simulink model "IdealGen_load_CtrlGen_wWT_abc_detailed"  (R2023b)
settings: Solver=VariableStepAuto  StartTime=0.0  StopTime=Tend  RelTol=1e-3
undefined symbols (not defined in the file): C_dc, c_drt, C_f, C_p_opt, f_nom, H_gen, H_vsm, H_WTR, I_dc_base, Ibase_hv, Ibase_lv, k_d_vsm, k_drt, k_p_p_vsm, k_p_q_vsm, K_pitch, Ki_cc, ki_q, Ki_vc, Kp_cc, Kp_vc, L_d, l_f, L_f, L_grid, L_mv, L_q, l_t_hvmv, l_t_mvlv, lambda_opt, Lbase1v, omega_nom, omega_WTR_min, omega_WTR_n, omega_WTR_sl, phase_shift_test_state, phase_shifts, pitch_max, pitch_min, Pitchanglevector, Pmax, Powercoefficient, psi_pm, R_a, r_f, R_grid, R_mv, r_t_hvmv, r_t_mvlv, R_WTR, rate_max, rate_min, rocof_slope, Rocof_test_state, Sbase1, Sbase_t1, T_base, T_pitch, T_servo, Tchange_gfm_ref ... (+12)
libraries: spsControlledVoltageSourceLib x6, slpidlib x6, spsPower3phInstantaneousLib x4, spsThreePhaseSeriesRLCBranchLib x4, spsCurrentMeasurementLib x3, spsThreePhaseVIMeasurementLib x3, spsRMSLib x3, spsabctodq0Lib x3, spsGroundLib x2, spsdq0toabcLib x2, spsSeriesRLCBranchLib x2, spsVoltageMeasurementLib x2
(part 1 of 2)
settings Model: Creator=s183702  LastModifiedBy=Martin Pedersen
settings HardwareCC: ProdBitPerLong=64  ProdLargestAtomicFloat=None  ProdHWDeviceType=AMD->Athlon 64

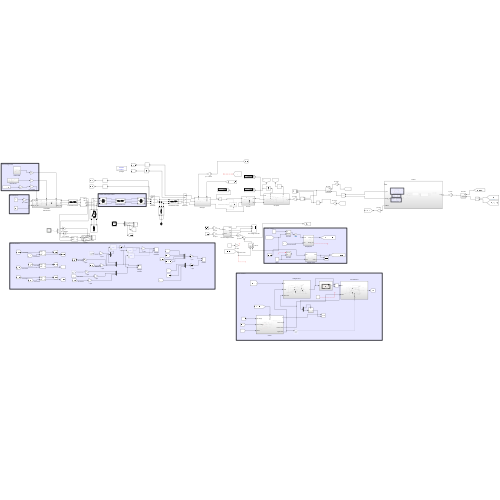
[thumbnail: Simulink's stored preview of the top-level diagram]
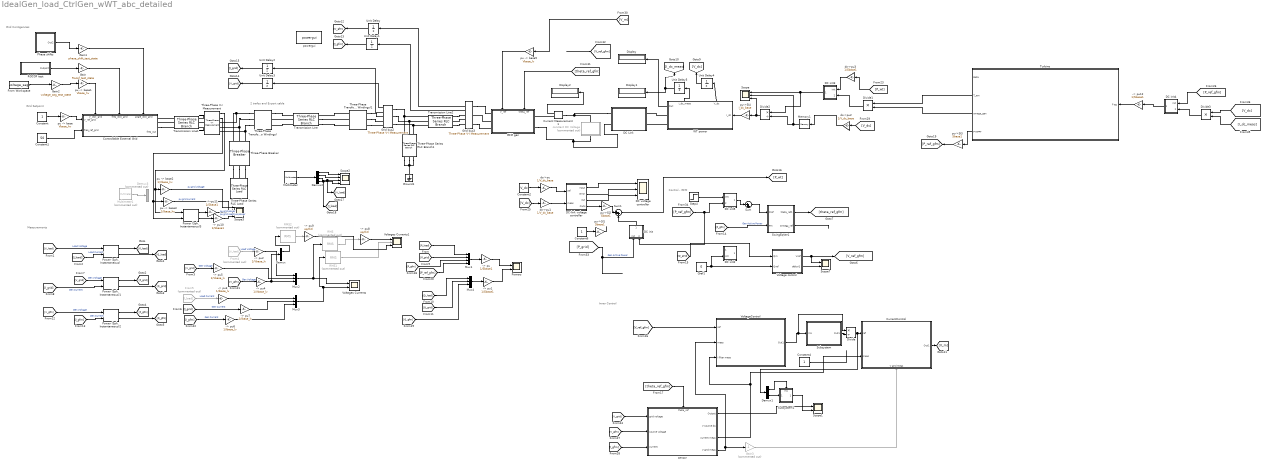
== system IdealGen_load_CtrlGen_wWT_abc_detailed ==
  note: Inner Control
  note: Grid Setpoint
  note: Grid Contigencies
  note: Control - GFM
  note: Measurements
  note: 2 trafos and Export cable
  -> pu{,1,10..12} (5 alike) : Gain  Gain=1/Sbase1
  -> pu2 : Gain  Gain=1/Vbase_lv
  -> pu3 : Gain  Gain=1/Ibase_lv
  -> pu4 : Gain  Gain=1/Vbase_lv
  -> pu5 : Gain  Gain=1/Vbase_lv
  -> pu6 : Gain  Gain=1/Ibase_lv
  -> pu7 : Gain  Gain=1/Ibase_lv
  -> pu8 : Gain  Gain=sqrt(2)
  -> pu9 : Gain  Gain=sqrt(2)
  Constant : Constant
  Constant1 : Constant  Value=50
  Constant2 : Constant  Value=V_dc
  Constant4 : Constant
  Constant6 : Constant
  Controllable External Grid : Subsystem
      settings: PortSchema="{\"entries\":[{\"content\":{\"sides\":[{\"content\":{\"connectorIds\":[\"In1\",\"In2\"]},\"type\":\"ConnectorPlacement.EquallySpacedRectSide\",\"uuid\":\"c82e3ee4-47de-4631-9682-a189e406d2fd\"},{\"content\":{\"connectorIds\":[\"RConn1\",\"RConn2\",\"RConn3\",\"Out1\"],\"side\":\"RIGHT\"},\"type\":\"ConnectorPlacement.EquallySpacedRectSide\",\"uuid\":\"b806e225-811d-4112-8c3d-45e9b8086e84\"},{\"content\":{\"connectorIds\":[\"In3\",\"In4\",\"In5\"],\"side\":\"TOP\"},\"type\":\"ConnectorPlacement.EquallySpacedRectSide\",\"uuid\":\"c79b677b-bc74-4454-b0f0-10f0f27e0767\"}]},\"type\":\"ConnectorPlacement.EquallySpacedConnector\",\"uuid\":\"44354c03-b4f0-403a-803b-b669dc1296a6\"}],\"packageUris\":[\"http://schema.mathworks.com/mf0/Connector/R2020b\"],\"version\":\"1.0\"}"
  Current Measurement1 : spsCurrentMeasurementLib/Current Measurement  PhasorSimulation=off  OutputType=Complex  PSBequivalent=0
  CurrentControl : Subsystem
      settings: PortSchema="{\"entries\":[{\"content\":{\"sides\":[{\"content\":{\"connectorIds\":[\"In1\",\"In2\"]},\"type\":\"ConnectorPlacement.EquallySpacedRectSide\",\"uuid\":\"219db9ea-637c-42c0-b87e-0a8373949a2f\"},{\"content\":{\"connectorIds\":[\"Out1\"],\"side\":\"RIGHT\"},\"type\":\"ConnectorPlacement.EquallySpacedRectSide\",\"uuid\":\"817edf77-a627-4761-8536-4c41ccdce557\"},{\"content\":{\"side\":\"TOP\"},\"type\":\"ConnectorPlacement.EquallySpacedRectSide\",\"uuid\":\"b4d64eff-9104-48e3-a4e2-ec81b224adc3\"},{\"content\":{\"connectorIds\":[\"In3\"],\"side\":\"BOTTOM\"},\"type\":\"ConnectorPlacement.EquallySpacedRectSide\",\"uuid\":\"8db682a6-86bb-4d51-9cc3-8f643a502240\"}]},\"type\":\"ConnectorPlacement.EquallySpacedConnector\",\"uuid\":\"cfbf309f-cee6-401c-8c28-748b4359d9c9\"}],\"packageUris\":[\"http://schema.mathworks.com/mf0/Connector/R2020b\"],\"version\":\"1.0\"}"
  DC Link : Subsystem
  DC init : Subsystem
  DC init2 : Subsystem
  DC init3 : Subsystem
  DC init4 : Subsystem
  DC init5 : Subsystem
  DC voltage controller : Scope  NumInputPorts=3
  DC-link voltage controller : Subsystem
  Demux : Demux  Outputs=3
  Demux1 : Demux  Outputs=2
  Demux2 : Demux
  Demux3 : Demux  Commented=on  Outputs=2
  Display : Display
  Display1 : Display
  Display2 : Display
  Divide : Product  Inputs=*/
  Divide1 : Product  Inputs=**
  Divide2 : Product  Inputs=*/
  Divide3 : Product  Inputs=**
  From Workspace : FromWorkspace  VariableName=voltage_sags
  From4 : From  Commented=on  GotoTag=V_load  TagVisibility=global
  From5 : From  Commented=on  GotoTag=I_load
  GFM gen : Subsystem
      settings: PortSchema="{\"entries\":[{\"content\":{\"sides\":[{\"content\":{\"connectorIds\":[\"LConn1\",\"LConn2\"]},\"type\":\"ConnectorPlacement.EquallySpacedRectSide\",\"uuid\":\"b9b898d8-aa2c-4fc0-879f-33950e845205\"},{\"content\":{\"connectorIds\":[\"RConn1\",\"RConn2\",\"RConn3\"],\"side\":\"RIGHT\"},\"type\":\"ConnectorPlacement.EquallySpacedRectSide\",\"uuid\":\"0f5f2870-ceda-40eb-961f-274893a00dd5\"},{\"content\":{\"connectorIds\":[\"In1\",\"In2\"],\"side\":\"TOP\"},\"type\":\"ConnectorPlacement.EquallySpacedRectSide\",\"uuid\":\"16b0f3cd-2bcf-4c98-bcc9-1e9131637ccf\"}]},\"type\":\"ConnectorPlacement.EquallySpacedConnector\",\"uuid\":\"5f5ec50b-7fca-4ced-b434-e49ba9676af4\"}],\"packageUris\":[\"http://schema.mathworks.com/mf0/Connector/R2020b\"],\"version\":\"1.0\"}"
  Gain : Gain  Gain=Rocof_test_state
  Gain1 : Gain  Gain=phase_shift_test_state
  Gain2 : Gain  Gain=voltage_sag_test_state
  Gain3 : Gain  Commented=on  Gain=-1
  Grid bus2 : spsThreePhaseVIMeasurementLib/Three-Phase V-I Measurement  VoltageMeasurement=phase-to-ground  SetLabelV=off  LabelV=V_grid  Vpu=off  VpuLL=off  CurrentMeasurement=yes  SetLabelI=off  LabelI=I_grid  Ipu=off  Pbase=100e6  Vbase=500e3  OutputType=Complex  PhasorSimulation=off  PSBequivalent=0
  Grid bus3 : spsThreePhaseVIMeasurementLib/Three-Phase V-I Measurement  VoltageMeasurement=phase-to-ground  SetLabelV=off  LabelV=V_gfm  Vpu=off  VpuLL=off  CurrentMeasurement=yes  SetLabelI=off  LabelI=I_gfm  Ipu=off  Pbase=100e6  Vbase=500e3  OutputType=Complex  PhasorSimulation=off  PSBequivalent=0
  Ground1 : spsGroundLib/Ground  LConnTagsString=a
  Memory1 : Memory  InitialCondition=1
  Multimeter : spsMultimeterLib/Multimeter  L=21  sel=[7 8 9 19 20 21 4 5 6 16 17 18]  yselected={}  Gain=[1 1 1 1 1 1 1 1 1 1 1 1]  OutputType=Complex  PlotAtSimulationStop=off  PhasorSimulation=off
  Multimeter1 : spsMultimeterLib/Multimeter  Commented=on  L=21  sel=[7 8 9 13 14 15]  yselected={}  Gain=[1 1 1 1 1 1]  OutputType=Complex  PlotAtSimulationStop=off  PhasorSimulation=off
  Mux1 : Mux
  Mux2 : Mux  Inputs=3
  Mux3 : Mux  Inputs=3
  Mux4 : Mux  Inputs=3
  Phase shifts : Subsystem
  Power (3ph, Instantaneous){,1..3} (4 alike) : spsPower3phInstantaneousLib/Power (3ph, Instantaneous)
  Powers : Scope  NumInputPorts=2
  Qref1 : Constant  Value=0
  RMS : spsRMSLib/RMS  Commented=on  TrueRMS=on  Freq=50  RMSInit=1  Ts=0
  RMS1 : spsRMSLib/RMS  Commented=on  TrueRMS=on  Freq=50  RMSInit=1  Ts=0
  RMS2 : spsRMSLib/RMS  Commented=on  TrueRMS=on  Freq=50  RMSInit=1  Ts=0
  ROCOF test : Subsystem
  Scope : Scope  NumInputPorts=3
  Scope1 : Scope  NumInputPorts=2
  Scope2 : Scope  NumInputPorts=4
  Scope3 : Scope  NumInputPorts=4
  Scope7 : Scope  NumInputPorts=2
  Step4 : Step  Time=Tchange_gfm_ref  Before=Sbase1*0.4  After=Sbase1*0.4  SampleTime=0
  Subsystem : Subsystem
  Subsystem1 : Subsystem
      settings: PortSchema="{\"entries\":[{\"content\":{\"sides\":[{\"content\":{\"connectorIds\":[\"In1\"]},\"type\":\"ConnectorPlacement.EquallySpacedRectSide\",\"uuid\":\"4a76dc79-b416-43cf-afab-f92cfdf0ce39\"},{\"content\":{\"connectorIds\":[\"Out1\"],\"side\":\"RIGHT\"},\"type\":\"ConnectorPlacement.EquallySpacedRectSide\",\"uuid\":\"95d72f6b-ef09-433d-aae0-c8341f391507\"},{\"content\":{\"connectorIds\":[\"In2\"],\"side\":\"TOP\"},\"type\":\"ConnectorPlacement.EquallySpacedRectSide\",\"uuid\":\"0145e476-49d1-4b43-865a-36bbad1700d0\"}]},\"type\":\"ConnectorPlacement.EquallySpacedConnector\",\"uuid\":\"1d1114a5-8d57-4d93-ab19-43d07f54280a\"}],\"packageUris\":[\"http://schema.mathworks.com/mf0/Connector/R2020b\"],\"version\":\"1.0\"}"
  Sum : Sum  Inputs=|++
  Sum1 : Sum  Inputs=|++
  SwingEqVer1 : Subsystem
  Three-Phase Series RLC Branch1 : spsThreePhaseSeriesRLCBranchLib/Three-Phase Series RLC Branch  LConnTagsString=A|B|C  RConnTagsString=A|B|C  BranchType=C  Resistance=0.001*Zbase1v  Inductance=L_f  Capacitance=C_f  Measurements=Branch currents
  Three-Phase Series RLC Load : spsThreePhaseSeriesRLCLoadLib/Three-Phase Series RLC Load  LConnTagsString=A|B|C  Configuration=Y (grounded)  NominalVoltage=Vbase_hv*sqrt(3/2)  Vabc=[1e3 1e3 1e3]  Vabcp=[1e3 1e3 1e3]  NominalFrequency=50  UnbalancedPower=off  ActivePower=Sbase1*0.5  InductivePower=0  CapacitivePower=0  Pabc=[10e3 9e3 11e3]  QLabc=[100 90 110]  QCabc=[100 90 110]  Pabcp=[10e3 9e3 11e3]  QLabcp=[100 90 110]  QCabcp=[100 90 110]  Measurements=Branch voltages and currents  LoadType=constant Z
  Three-Phase Transformer (Two Windings) : spsThreePhaseTransformerTwoWindingsLib/Three-Phase Transformer (Two Windings)  Winding1Connection=Yg  Winding2Connection=Yg  CoreType=Three single-phase transformers  SetSaturation=off  Hysteresis=off  DataFile='hysteresis'  SetInitialFlux=off  Measurements=None  UNITS=pu  NominalPower=[ Sbase1 , f_nom ]  Winding1=[ Vbase_hv*sqrt(3/2) , r_t_hvmv/2 , l_t_hvmv/2]  Winding2=[ Vbase_mv*sqrt(3/2) , r_t_hvmv/2, l_t_hvmv/2 ]  Rm=500  Lm=500  L0=0.5  Saturation=[ 0,0 ; 0.0024,1.2 ; 1.0,1.52 ]  InitialFluxes=[ 0.8 , -0.8 , 0.7 ]  BreakLoop=off  DiscreteSolver=Trapezoidal iterative  DataType=off  TransfoNumber=1
  Three-Phase Transformer (Two Windings)1 : spsThreePhaseTransformerTwoWindingsLib/Three-Phase Transformer (Two Windings)  Winding1Connection=Yg  Winding2Connection=Yg  CoreType=Three single-phase transformers  SetSaturation=off  Hysteresis=off  DataFile='hysteresis'  SetInitialFlux=off  Measurements=None  UNITS=pu  NominalPower=[ Sbase_t1 , f_nom ]  Winding1=[ Vbase_mv*sqrt(3/2) , r_t_mvlv/2 , l_t_mvlv/2]  Winding2=[ Vbase_lv*sqrt(3/2) , r_t_mvlv/2, l_t_mvlv/2 ]  Rm=500  Lm=500  L0=0.5  Saturation=[ 0,0 ; 0.0024,1.2 ; 1.0,1.52 ]  InitialFluxes=[ 0.8 , -0.8 , 0.7 ]  BreakLoop=off  DiscreteSolver=Trapezoidal iterative  DataType=off  TransfoNumber=1
  Three-Phase V-I Measurement : spsThreePhaseVIMeasurementLib/Three-Phase V-I Measurement  VoltageMeasurement=phase-to-ground  SetLabelV=off  LabelV=Vabc  Vpu=off  VpuLL=off  CurrentMeasurement=yes  SetLabelI=off  LabelI=Iabc  Ipu=off  Pbase=100e6  Vbase=500e3  OutputType=Complex  PhasorSimulation=off  PSBequivalent=0
  Three-Phase Breaker : spsThreePhaseBreakerLib/Three-Phase Breaker  InitialState=open  SwitchA=on  SwitchB=on  SwitchC=on  SwitchTimes=[30]  External=off  BreakerResistance=0.01  SnubberResistance=1e6  SnubberCapacitance=inf  Measurements=Breaker voltages and currents
  Transmission Line : spsThreePhaseSeriesRLCBranchLib/Three-Phase Series RLC Branch  LConnTagsString=A|B|C  RConnTagsString=A|B|C  BranchType=RL  Resistance=R_mv  Inductance=L_mv  Capacitance=0  Measurements=None
  Transmission Line1 : spsThreePhaseSeriesRLCBranchLib/Three-Phase Series RLC Branch  LConnTagsString=A|B|C  RConnTagsString=A|B|C  BranchType=RL  Resistance=R_grid  Inductance=L_grid  Capacitance=0  Measurements=Branch voltages and currents
  Transmission Line2 : spsThreePhaseSeriesRLCBranchLib/Three-Phase Series RLC Branch  LConnTagsString=A|B|C  RConnTagsString=A|B|C  BranchType=RL  Resistance=r_f*Zbase1v  Inductance=l_f*Lbase1v  Capacitance=0  Measurements=None
  Turbine : Subsystem
  Unit Delay{,1..3,5} (5 alike) : UnitDelay  SampleTime=-1  HasFrameUpgradeWarning=on
  Unit Delay4 : UnitDelay  InitialCondition=V_dc  SampleTime=-1  HasFrameUpgradeWarning=on
  Voltage control : Subsystem
  VoltageControl : Subsystem
  Voltages Currents : Scope  NumInputPorts=2
  Voltages Currents1 : Scope  NumInputPorts=3
  WT power : Subsystem
      settings: PortSchema="{\"entries\":[{\"content\":{\"sides\":[{\"content\":{\"connectorIds\":[\"In1\"]},\"type\":\"ConnectorPlacement.EquallySpacedRectSide\",\"uuid\":\"9d3e38d2-6add-483d-9a31-3b5598dff8d3\"},{\"content\":{\"connectorIds\":[\"Out1\",\"RConn1\",\"RConn2\"],\"side\":\"RIGHT\"},\"type\":\"ConnectorPlacement.EquallySpacedRectSide\",\"uuid\":\"7ce5d226-07b0-4d85-bacd-eba224635451\"},{\"content\":{\"connectorIds\":[\"Out2\",\"Out3\"],\"side\":\"TOP\"},\"type\":\"ConnectorPlacement.EquallySpacedRectSide\",\"uuid\":\"1864accd-580c-4e01-b41e-4bc1921d0b77\"},{\"content\":{\"side\":\"BOTTOM\"},\"type\":\"ConnectorPlacement.EquallySpacedRectSide\",\"uuid\":\"0a771f6d-f5fb-412d-b2d7-9d95c39f39de\"}]},\"type\":\"ConnectorPlacement.EquallySpacedConnector\",\"uuid\":\"874bd654-abb7-47d1-80fe-1eaf36f4fe8a\"}],\"packageUris\":[\"http://schema.mathworks.com/mf0/Connector/R2020b\"],\"version\":\"1.0\"}"
  constant DC Voltage : Subsystem  Commented=on
  dc->pu : Gain  Gain=1/V_dc_base
  dc->pu1 : Gain  Gain=1/V_dc_base
  dc->pu2 : Gain  Gain=1/V_dc_base
  dc->pu3 : Gain  Gain=1/Sbase1
  powergui : sps_lib/powergui  Priority=1  SimulationMode=Discrete  SampleTime=5e-6  frequency=60  Iterations=50  frequencyindice=0  Pbase=100e6  ErrMax=1e-4  UnitsV=kV  UnitsW=MW  buscounter=0  FunctionMessages=off  echomessages=off  EnableUseOfTLC=off  CurrentSourceSwitches=off  DisableSnubberDevices=off  DisableRonSwitches=off  DisableVfSwitches=off  DisplayEquations=off  AutomaticDiscreteSolvers=off  SolverType=Tustin/Backward Euler (TBE)  Interpol=off  ExternalGateDelay=off  methode=off  Ts=100  x0status=blocks  SPID=on  SwTol=0  HookPort=off  NonlinearTolerance=1e-4  nMaxIteration=100  ContinueOnMaxIteration=off  RestoreLinks=warning  ResistiveCurrentMeasurement=off  Frange=[0:2:500]  Ylog=off  Xlog=on  ShowGrid=off  save=off  variable=ZData  structure=0  ZoomFFT=off  StartTime=0.0  cycles=1  DisplayStyle=1  fundamental=60  FreqAxis=off  MaxFrequency=1000  frequencyindicesteady=1  RmsSteady=1  display=off
  "pu -> base" : Gain  Gain=Vbase_hv
  "pu -> base1" : Gain  Gain=Vbase_hv
  "pu -> base2" : Gain  Gain=1/Vbase_hv
  "pu -> base3" : Gain  Gain=1/Ibase_hv
  "pu -> base5" : Gain  Gain=Vbase_lv
  pu->SI1 : Gain  Gain=Sbase1
  pu->SI2 : Gain  Gain=Sbase1
  pu->SI3 : Gain  Gain=Sbase1
  pu->SI4 : Gain  Gain=I_dc_base
  sensor : Subsystem
      settings: PortSchema="{\"entries\":[{\"content\":{\"sides\":[{\"content\":{\"connectorIds\":[\"In1\",\"In2\",\"In3\"]},\"type\":\"ConnectorPlacement.EquallySpacedRectSide\",\"uuid\":\"f6076434-f402-4e41-b507-98b228e724d5\"},{\"content\":{\"connectorIds\":[\"Out1\",\"Out2\",\"Out3\",\"Out4\"],\"side\":\"RIGHT\"},\"type\":\"ConnectorPlacement.EquallySpacedRectSide\",\"uuid\":\"ad78b019-92bf-45d4-be49-d5eeb6323d07\"},{\"content\":{\"side\":\"TOP\"},\"type\":\"ConnectorPlacement.EquallySpacedRectSide\",\"uuid\":\"9dc9234e-7a1d-4b97-8830-6d3adbb504ce\"},{\"content\":{\"connectorIds\":[\"In4\"],\"side\":\"BOTTOM\"},\"type\":\"ConnectorPlacement.EquallySpacedRectSide\",\"uuid\":\"085a8b4b-0a39-42f8-9e4d-5287113458ab\"}]},\"type\":\"ConnectorPlacement.EquallySpacedConnector\",\"uuid\":\"c1a424bf-dbfe-42ba-bd00-ed441f443675\"}],\"packageUris\":[\"http://schema.mathworks.com/mf0/Connector/R2020b\"],\"version\":\"1.0\"}"
  wires:
  From5/1 -> -> pu3/1  "Load Current"
  From4/1 -> -> pu2/1  "Load Voltage"
  [V_grid] -> -> pu5/1  "Gen Voltage"
  [I_grid] -> -> pu7/1  "Gen Current"
  "pu -> base"/1 -> Controllable External Grid/1(V_ref_grid)
  Constant/1 -> "pu -> base"/1
  Constant1/1 -> Controllable External Grid/2(freq_ref_grid)
  Gain2/1 -> "pu -> base1"/1
  ROCOF test/1(Outport) -> Gain/1
  "pu -> base1"/1 -> Controllable External Grid/3(V_dist_grid)
  [V_load] -> "Power (3ph, Instantaneous)"/1  "Load Voltage"
  [I_load] -> "Power (3ph, Instantaneous)"/2  "Load Current"
  [V_grid] -> "Power (3ph, Instantaneous)1"/1  "Gen Voltage"
  [I_grid] -> "Power (3ph, Instantaneous)1"/2  "Gen Current"
  "Power (3ph, Instantaneous)"/1 -> [P_load]
  "Power (3ph, Instantaneous)"/2 -> [Q_load]
  "Power (3ph, Instantaneous)1"/1 -> [P_grid]
  "Power (3ph, Instantaneous)1"/2 -> [Q_grid]
  [Q_load] -> Mux4/1
  [Q_grid] -> Mux4/2
  [P_grid] -> Mux1/2
  [P_load] -> Mux1/1
  Mux4/1 -> -> pu1/1
  Mux1/1 -> -> pu/1
  -> pu/1 -> Powers/1
  -> pu1/1 -> Powers/2
  "pu -> base5"/1 -> GFM gen/2(V_ref)
  "Power (3ph, Instantaneous)2"/2 -> [Q_gfm]
  "Power (3ph, Instantaneous)2"/1 -> [P_gfm]
  [I_gfm] -> "Power (3ph, Instantaneous)2"/2  "Gen Current"
  [V_gfm] -> "Power (3ph, Instantaneous)2"/1  "Gen Voltage"
  [P_gfm] -> SwingEqVer1/2(Pm)  "Gen Active Power"
  SwingEqVer1/2(Omega_ref) -> ?
  SwingEqVer1/1(theta_ref1) -> [theta_ref_gfm]
  Qref1/1 -> DC init2/2(init), Voltage control/2(Qref)
  Voltage control/1(Vref) -> Scope7/1, [V_ref_gfm]
  Voltage control/2(delta Q) -> Scope7/2
  ? -> DC init2/1(second)
  [V_ref_gfm] -> ?
  [theta_ref_gfm] -> GFM gen/1(theta_ref)
  [P_gfm] -> Mux1/3
  [Q_gfm] -> Mux4/3
  [P_ref_gfm] -> Mux1/4
  [V_gfm] -> -> pu4/1  "Gen Voltage"
  [I_gfm] -> -> pu6/1  "Gen Current"
  Mux2/1 -> RMS/1, Voltages Currents/1
  Mux3/1 -> RMS1/1, Voltages Currents/2
  -> pu2/1 -> Mux2/1
  -> pu4/1 -> Demux/1, Mux2/3
  -> pu5/1 -> Mux2/2
  -> pu3/1 -> Mux3/1
  -> pu6/1 -> Mux3/3
  RMS/1 -> -> pu8/1
  RMS1/1 -> Voltages Currents1/2
  -> pu7/1 -> Mux3/2
  -> pu8/1 -> Voltages Currents1/1
  RMS2/1 -> -> pu9/1
  -> pu9/1 -> Voltages Currents1/3
  Demux/1 -> RMS2/1
  WT power/2(V_dc) -> Unit Delay4/1
  WT power/1(Pwt) -> Display/1
  Constant2/1 -> dc->pu/1
  [V_dc] -> dc->pu1/1
  DC-link voltage controller/1(input) -> DC voltage controller/1
  DC-link voltage controller/2(error) -> DC voltage controller/2
  DC-link voltage controller/3(out) -> DC voltage controller/3
  WT power/3(i_dc_meas) -> Unit Delay5/1
  Divide1/1 -> DC init3/2(second)
  Memory1/1 -> Scope/2, Divide2/2
  Divide2/1 -> Scope/3, pu->SI4/1
  dc->pu/1 -> DC-link voltage controller/1(ref)
  dc->pu1/1 -> DC-link voltage controller/2(meas)
  Gain/1 -> Controllable External Grid/4(freq_dist_grid)
  Gain1/1 -> Controllable External Grid/5(angle_dist_grid)
  Phase shifts/1(Out2) -> Gain1/1
  From Workspace/1 -> Gain2/1
  [theta_ref_gfm] -> sensor/4(theta_ref)
  [V_ref_gfm] -> VoltageControl/1(ref)
  sensor/1(V grid meas) -> VoltageControl/2(meas), Gain3/1
  sensor/2(current meas) -> VoltageControl/3(I filter meas), CurrentControl/2(meas)
  [I_gfm] -> sensor/1(current)
  [V_grid] -> sensor/3(grid voltage)
  [V_gfm] -> sensor/2(source voltage)
  CurrentControl/1(Out1) -> [V_m]
  [V_m] -> "pu -> base5"/1
  Gain3/1 -> CurrentControl/3(V grid meas)
  Divide/1 -> Demux1/1, CurrentControl/1(ref)
  VoltageControl/1(Out1) -> Divide/1, Subsystem/1(In1)
  Constant4/1 -> ?
  Grid bus3/1 -> Unit Delay/1
  Unit Delay2/1 -> [I_grid]
  Unit Delay3/1 -> [V_grid]
  Unit Delay1/1 -> [I_gfm]
  Unit Delay/1 -> [V_gfm]
  Grid bus3/2 -> Unit Delay1/1
  Grid bus2/1 -> Unit Delay3/1
  Grid bus2/2 -> Unit Delay2/1
  Unit Delay4/1 -> [V_dc]
  Unit Delay5/1 -> [I_dc_meas], Display1/1
  [V_dc] -> dc->pu2/1
  Sum/1 -> SwingEqVer1/1(Pref)
  Constant6/1 -> pu->SI1/1
  DC-link voltage controller/4(Out4) -> pu->SI2/1
  [P_grid] -> DC init/1(init)  "Gen Active Power"
  pu->SI2/1 -> Sum1/1
  Subsystem/1(Out1) -> Divide/2
  pu->SI1/1 -> ?
  sensor/4(Output) -> Scope1/1
  Subsystem1/1(Out1) -> Scope1/2
  Demux1/1 -> Subsystem1/2(In1)
  Demux1/2 -> Subsystem1/1(In2)
  Multimeter/1 -> Demux2/1
  Demux2/1 -> Scope2/1
  Demux2/2 -> Scope2/2
  Demux2/3 -> Scope2/3, [V_load]
  Demux2/4 -> [I_load], Scope2/4
  Multimeter1/1 -> Demux3/1
  Three-Phase V-I Measurement/1 -> "Power (3ph, Instantaneous)3"/1, "pu -> base2"/1
  "pu -> base2"/1 -> Scope3/1  "pu grid voltage"
  Three-Phase V-I Measurement/2 -> "Power (3ph, Instantaneous)3"/2, "pu -> base3"/1
  "pu -> base3"/1 -> Scope3/2  "pu grid current"
  "Power (3ph, Instantaneous)3"/2 -> -> pu10/1
  "Power (3ph, Instantaneous)3"/1 -> -> pu11/1
  -> pu11/1 -> Scope3/3  "pu grid power"
  -> pu10/1 -> Scope3/4  "pu grid reactive power"
  Turbine/4(P MPPT) -> pu->SI3/1
  pu->SI3/1 -> [P_ref_gfm]
  Turbine/3(omega_gen) -> Divide1/2
  [P_ref_gfm] -> DC init4/1(init)
  -> pu12/1 -> Turbine/1(P ag)
  Turbine/2(T_em) -> Divide1/1
  dc->pu2/1 -> Memory1/1
  pu->SI4/1 -> WT power/1(I_dc)
  Divide3/1 -> DC init4/2(second)
  [I_dc_meas] -> Divide3/2
  DC init3/1("   ") -> Divide2/1, Scope/1
  Current Measurement1/1 -> Display2/1
  [Q_grid] -> Voltage control/1(Qm)
  [P_ref_gfm] -> DC init5/2(second), DC init/2(second)
  Sum1/1 -> [P_wt]
  DC init4/1("   ") -> -> pu12/1
  [V_dc] -> Divide3/1
  [P_wt] -> dc->pu3/1
  DC init5/1("   ") -> Sum/1
  Step4/1 -> DC init5/1(init)
  dc->pu3/1 -> DC init3/1(init)
  DC init/1("   ") -> Sum1/2
  connections:
  Three-Phase Series RLC Branch1/LConn2 -- Grid bus2/LConn2 -- Transmission Line2/LConn2
  Three-Phase Series RLC Branch1/LConn1 -- Grid bus2/LConn1 -- Transmission Line2/LConn1
  Three-Phase Series RLC Branch1/LConn3 -- Grid bus2/LConn3 -- Transmission Line2/LConn3
  Three-Phase Transformer (Two Windings)1/RConn1 -- Grid bus2/RConn1
  Three-Phase Transformer (Two Windings)1/RConn2 -- Grid bus2/RConn2
  Three-Phase Transformer (Two Windings)1/RConn3 -- Grid bus2/RConn3
  Transmission Line1/LConn1 -- Controllable External Grid/RConn1
  Transmission Line1/LConn2 -- Controllable External Grid/RConn2
  Controllable External Grid/RConn3 -- Transmission Line1/LConn3
  GFM gen/RConn2 -- Grid bus3/LConn2
  Grid bus3/LConn1 -- GFM gen/RConn1
  Grid bus3/LConn3 -- GFM gen/RConn3
  Transmission Line2/RConn1 -- Grid bus3/RConn1
  Grid bus3/RConn2 -- Transmission Line2/RConn2
  Transmission Line2/RConn3 -- Grid bus3/RConn3
  GFM gen/LConn2 -- DC Link/LConn2 -- constant DC Voltage/RConn1
  WT power/RConn1 -- DC Link/RConn1
  WT power/RConn2 -- DC Link/RConn2
  Three-Phase Series RLC Branch1/RConn2 -- Three-Phase Series RLC Branch1/RConn1 -- Three-Phase Series RLC Branch1/RConn3 -- Ground1/LConn1
  Three-Phase Transformer (Two Windings)/RConn1 -- Transmission Line/LConn1
  Transmission Line/RConn2 -- Three-Phase Transformer (Two Windings)1/LConn2
  Transmission Line/LConn2 -- Three-Phase Transformer (Two Windings)/RConn2
  Transmission Line/RConn3 -- Three-Phase Transformer (Two Windings)1/LConn3
  Three-Phase Transformer (Two Windings)1/LConn1 -- Transmission Line/RConn1
  Transmission Line/LConn3 -- Three-Phase Transformer (Two Windings)/RConn3
  Three-Phase Transformer (Two Windings)/LConn1 -- Three-Phase V-I Measurement/RConn1 -- Three-Phase Breaker/LConn1
  Three-Phase Transformer (Two Windings)/LConn2 -- Three-Phase V-I Measurement/RConn2 -- Three-Phase Breaker/LConn2
  Three-Phase Transformer (Two Windings)/LConn3 -- Three-Phase V-I Measurement/RConn3 -- Three-Phase Breaker/LConn3
  DC Link/LConn1 -- constant DC Voltage/LConn1 -- Current Measurement1/LConn1
  Three-Phase Breaker/RConn1 -- Three-Phase Series RLC Load/LConn1
  Three-Phase Breaker/RConn2 -- Three-Phase Series RLC Load/LConn2
  Three-Phase Breaker/RConn3 -- Three-Phase Series RLC Load/LConn3
  Three-Phase V-I Measurement/LConn2 -- Transmission Line1/RConn2
  Three-Phase V-I Measurement/LConn1 -- Transmission Line1/RConn1
  Three-Phase V-I Measurement/LConn3 -- Transmission Line1/RConn3
  Current Measurement1/RConn1 -- GFM gen/LConn1

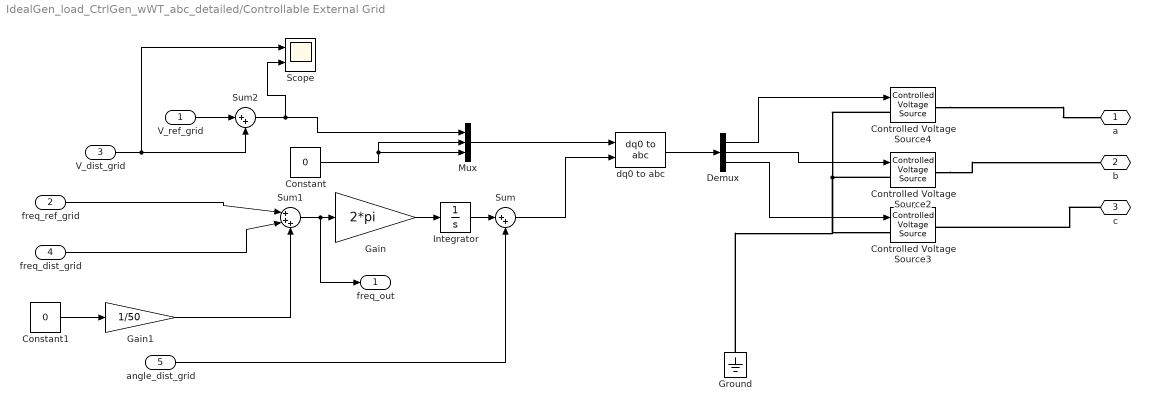
== system IdealGen_load_CtrlGen_wWT_abc_detailed/Controllable External Grid ==
  V_ref_grid : Inport
  freq_ref_grid : Inport  Port=2
  V_dist_grid : Inport  Port=3
  freq_dist_grid : Inport  Port=4
  angle_dist_grid : Inport  Port=5
  Constant : Constant  Value=0
  Constant1 : Constant  Value=0
  Controlled Voltage Source2 : spsControlledVoltageSourceLib/Controlled Voltage Source  Initialize=on  Source_Type=AC  Amplitude=Vbase_lv  Phase=-120  Frequency=50  Measurements=None
  Controlled Voltage Source3 : spsControlledVoltageSourceLib/Controlled Voltage Source  Initialize=on  Source_Type=AC  Amplitude=Vbase_lv  Phase=120  Frequency=50  Measurements=None
  Controlled Voltage Source4 : spsControlledVoltageSourceLib/Controlled Voltage Source  Initialize=on  Source_Type=AC  Amplitude=Vbase_lv  Phase=0  Frequency=50  Measurements=None
  Demux : Demux  Outputs=3
  Gain : Gain  Gain=2*pi
  Gain1 : Gain  Gain=1/50
  Ground : spsGroundLib/Ground  LConnTagsString=a
  Integrator : Integrator
  Mux : Mux  Inputs=3
  Scope : Scope  NumInputPorts=2
  Sum : Sum  Inputs=|++
  Sum1 : Sum  Inputs=|+++
  Sum2 : Sum  Inputs=|++
  dq0 to abc : spsdq0toabcLib/dq0 to abc  Alignment=90 degrees behind phase A axis
  a : PMIOPort  Side=Right
  b : PMIOPort  Port=2  Side=Right
  c : PMIOPort  Port=3  Side=Right
  freq_out : Outport
  wires:
  Demux/1 -> Controlled Voltage Source4/1
  Demux/2 -> Controlled Voltage Source2/1
  Demux/3 -> Controlled Voltage Source3/1
  Mux/1 -> dq0 to abc/1
  Constant/1 -> Mux/2, Mux/3
  dq0 to abc/1 -> Demux/1
  Sum2/1 -> Scope/2, Mux/1
  Gain/1 -> Integrator/1
  Integrator/1 -> Sum/1
  angle_dist_grid/1 -> Sum/2
  freq_dist_grid/1 -> Sum1/2
  Sum1/1 -> freq_out/1, Gain/1
  freq_ref_grid/1 -> Sum1/1
  Sum/1 -> dq0 to abc/2
  V_ref_grid/1 -> Sum2/1
  V_dist_grid/1 -> Sum2/2, Scope/1
  Gain1/1 -> Sum1/3
  Constant1/1 -> Gain1/1
  connections:
  Controlled Voltage Source2/LConn1 -- Controlled Voltage Source4/LConn1 -- Ground/LConn1 -- Controlled Voltage Source3/LConn1
  c/RConn1 -- Controlled Voltage Source3/RConn1
  Controlled Voltage Source4/RConn1 -- a/RConn1
  Controlled Voltage Source2/RConn1 -- b/RConn1

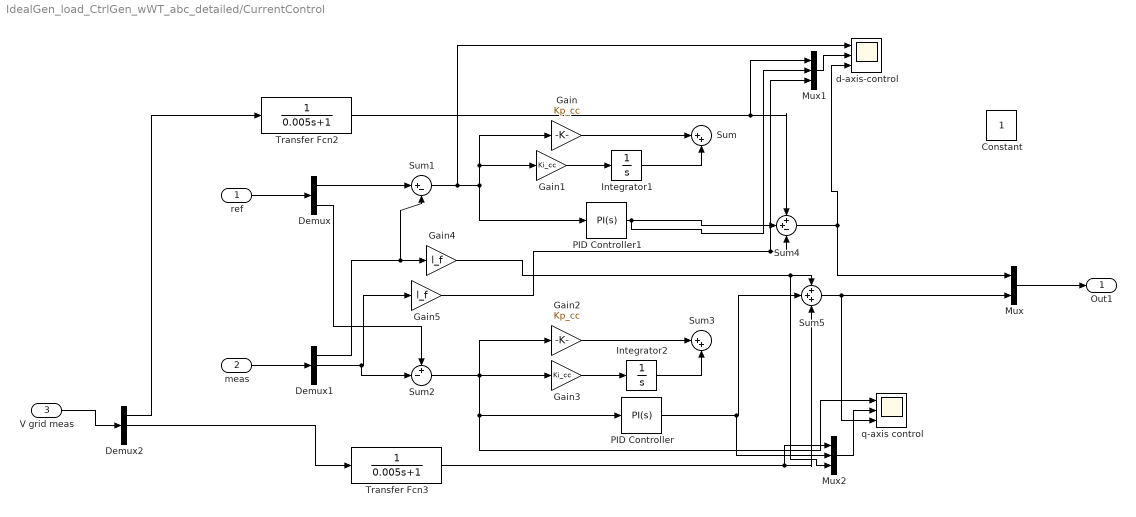
== system IdealGen_load_CtrlGen_wWT_abc_detailed/CurrentControl ==
  ref : Inport
  meas : Inport  Port=2
  V grid meas : Inport  Port=3
  Constant : Constant
  Demux : Demux  Outputs=2
  Demux1 : Demux  Outputs=3
  Demux2 : Demux  Outputs=3
  Gain : Gain  Gain=Kp_cc
  Gain1 : Gain  Gain=Ki_cc
  Gain2 : Gain  Gain=Kp_cc
  Gain3 : Gain  Gain=Ki_cc
  Gain4 : Gain  Gain=l_f
  Gain5 : Gain  Gain=l_f
  Integrator1 : Integrator
  Integrator2 : Integrator
  Mux : Mux  Inputs=2
  Mux1 : Mux  Inputs=3
  Mux2 : Mux  Inputs=3
  PID Controller : slpidlib/PID Controller  Controller=PI  Form=Parallel  TimeDomain=Continuous-time  UseExternalTs=off  SampleTime=-1  IntegratorMethod=Forward Euler  FilterMethod=Forward Euler  ControllerParametersSource=internal  P=Kp_cc  I=Ki_cc  UseKiTs=off  D=0  N=100  UseFilter=on  TunerSelectOption=Transfer Function Based (PID Tuner App)  InitialConditionSource=internal  InitialConditionForIntegrator=0  InitialConditionForFilter=0  DifferentiatorICPrevScaledInput=0  ExternalReset=none  TrackingMode=off  Kt=1  LimitOutput=off  SatLimitsSource=internal  UpperSaturationLimit=inf  LowerSaturationLimit=-inf  LinearizeAsGain=on  AntiWindupMode=none  Kb=1  LimitIntegrator=off  UpperIntegratorSaturationLimit=inf  LowerIntegratorSaturationLimit=-inf  POutMin=[]  POutMax=[]  IOutMin=[]  IOutMax=[]  DOutMin=[]  DOutMax=[]  NOutMin=[]  NOutMax=[]  SumOutMin=[]  SumOutMax=[]  SaturationOutMin=[]  SaturationOutMax=[]  PParamMin=[]  PParamMax=[]  IParamMin=[]  IParamMax=[]  DParamMin=[]  DParamMax=[]  NParamMin=[]  NParamMax=[]  KbParamMin=[]  KbParamMax=[]  KtParamMin=[]  KtParamMax=[]  KbOutMin=[]  KbOutMax=[]  KtOutMin=[]  KtOutMax=[]  IntegratorOutMin=[]  IntegratorOutMax=[]  FilterOutMin=[]  FilterOutMax=[]  SumI1OutMin=[]  SumI1OutMax=[]  SumI2OutMin=[]  SumI2OutMax=[]  SumI3OutMin=[]  SumI3OutMax=[]  SumI4OutMin=[]  SumI4OutMax=[]  SumDOutMin=[]  SumDOutMax=[]  DifferentiatorOutMin=[]  DifferentiatorOutMax=[]  FilterDiffOutCoefMin=[]  FilterDiffOutCoefMax=[]  ReciprocalOutMin=[]  ReciprocalOutMax=[]  SumDenOutMin=[]  SumDenOutMax=[]  SumNumOutMin=[]  SumNumOutMax=[]  DivideOutMin=[]  DivideOutMax=[]  UdiffTsProdOutMin=[]  UdiffTsProdOutMax=[]  NTsProdOutMin=[]  NTsProdOutMax=[]  UintegralTsProdOutMin=[]  UintegralTsProdOutMax=[]  UngainTsProdOutMin=[]  UngainTsProdOutMax=[]  ClampingZeroOutDataTypeStr=Inherit: Inherit via back propagation  ClampingZeroOutMin=[]  ClampingZeroOutMax=[]  FilterDenConstantOutDataTypeStr=Inherit: Inherit via back propagation  FilterDenConstantOutMin=[]  FilterDenConstantOutMax=[]  PCopyOutDataTypeStr=Inherit: Inherit via back propagation  PCopyOutMin=[]  PCopyOutMax=[]  NCopyOutDataTypeStr=Inherit: Inherit via back propagation  NCopyOutMin=[]  NCopyOutMax=[]  IntegratorContinuousStateAttributes=''  IntegratorStateMustResolveToSignalObject=off  IntegratorRTWStateStorageClass=Auto  FilterContinuousStateAttributes=''  FilterStateMustResolveToSignalObject=off  FilterRTWStateStorageClass=Auto  ParallelPVariant=InternalParameters  IdealPVariant=Disabled  IVariant=InternalParameters  DVariant=Disabled  IntegratorVariant=Continuous  SatVariant=Disabled  AWVariant=Passthrough  PCopyVariant=Disabled  TRVariant=Disabled  FdbkBlocksVariant=Forward  IdealPFdbkVariant=Disabled  SatFdbkVariant=Disabled  DerivativeFilterVariant=Disabled  NVariant=Disabled  NCopyVariant=Disabled_SignalSpec  FilterICVariant=Disabled  IntegratorICVariant=InternalICs  ExternalResetVariant=Disabled  TRSumVariant=Passthrough  SumFdbkVariant=Disabled  SumVariant=Sum_PI  TsampFilterVariant=InternalTs  TsampNgainVariant=Passthrough  TsampIntegralVariant=Disabled_SignalSpec  ExternalSaturationOutDataTypeStr=Inherit: Same as second input
  PID Controller1 : slpidlib/PID Controller  Controller=PI  Form=Parallel  TimeDomain=Continuous-time  UseExternalTs=off  SampleTime=-1  IntegratorMethod=Forward Euler  FilterMethod=Forward Euler  ControllerParametersSource=internal  P=Kp_cc  I=Ki_cc  UseKiTs=off  D=0  N=100  UseFilter=on  TunerSelectOption=Transfer Function Based (PID Tuner App)  InitialConditionSource=internal  InitialConditionForIntegrator=1  InitialConditionForFilter=0  DifferentiatorICPrevScaledInput=0  ExternalReset=none  TrackingMode=off  Kt=1  LimitOutput=off  SatLimitsSource=internal  UpperSaturationLimit=inf  LowerSaturationLimit=-inf  LinearizeAsGain=on  AntiWindupMode=none  Kb=1  LimitIntegrator=off  UpperIntegratorSaturationLimit=inf  LowerIntegratorSaturationLimit=-inf  POutMin=[]  POutMax=[]  IOutMin=[]  IOutMax=[]  DOutMin=[]  DOutMax=[]  NOutMin=[]  NOutMax=[]  SumOutMin=[]  SumOutMax=[]  SaturationOutMin=[]  SaturationOutMax=[]  PParamMin=[]  PParamMax=[]  IParamMin=[]  IParamMax=[]  DParamMin=[]  DParamMax=[]  NParamMin=[]  NParamMax=[]  KbParamMin=[]  KbParamMax=[]  KtParamMin=[]  KtParamMax=[]  KbOutMin=[]  KbOutMax=[]  KtOutMin=[]  KtOutMax=[]  IntegratorOutMin=[]  IntegratorOutMax=[]  FilterOutMin=[]  FilterOutMax=[]  SumI1OutMin=[]  SumI1OutMax=[]  SumI2OutMin=[]  SumI2OutMax=[]  SumI3OutMin=[]  SumI3OutMax=[]  SumI4OutMin=[]  SumI4OutMax=[]  SumDOutMin=[]  SumDOutMax=[]  DifferentiatorOutMin=[]  DifferentiatorOutMax=[]  FilterDiffOutCoefMin=[]  FilterDiffOutCoefMax=[]  ReciprocalOutMin=[]  ReciprocalOutMax=[]  SumDenOutMin=[]  SumDenOutMax=[]  SumNumOutMin=[]  SumNumOutMax=[]  DivideOutMin=[]  DivideOutMax=[]  UdiffTsProdOutMin=[]  UdiffTsProdOutMax=[]  NTsProdOutMin=[]  NTsProdOutMax=[]  UintegralTsProdOutMin=[]  UintegralTsProdOutMax=[]  UngainTsProdOutMin=[]  UngainTsProdOutMax=[]  ClampingZeroOutDataTypeStr=Inherit: Inherit via back propagation  ClampingZeroOutMin=[]  ClampingZeroOutMax=[]  FilterDenConstantOutDataTypeStr=Inherit: Inherit via back propagation  FilterDenConstantOutMin=[]  FilterDenConstantOutMax=[]  PCopyOutDataTypeStr=Inherit: Inherit via back propagation  PCopyOutMin=[]  PCopyOutMax=[]  NCopyOutDataTypeStr=Inherit: Inherit via back propagation  NCopyOutMin=[]  NCopyOutMax=[]  IntegratorContinuousStateAttributes=''  IntegratorStateMustResolveToSignalObject=off  IntegratorRTWStateStorageClass=Auto  FilterContinuousStateAttributes=''  FilterStateMustResolveToSignalObject=off  FilterRTWStateStorageClass=Auto  ParallelPVariant=InternalParameters  IdealPVariant=Disabled  IVariant=InternalParameters  DVariant=Disabled  IntegratorVariant=Continuous  SatVariant=Disabled  AWVariant=Passthrough  PCopyVariant=Disabled  TRVariant=Disabled  FdbkBlocksVariant=Forward  IdealPFdbkVariant=Disabled  SatFdbkVariant=Disabled  DerivativeFilterVariant=Disabled  NVariant=Disabled  NCopyVariant=Disabled_SignalSpec  FilterICVariant=Disabled  IntegratorICVariant=InternalICs  ExternalResetVariant=Disabled  TRSumVariant=Passthrough  SumFdbkVariant=Disabled  SumVariant=Sum_PI  TsampFilterVariant=InternalTs  TsampNgainVariant=Passthrough  TsampIntegralVariant=Disabled_SignalSpec  ExternalSaturationOutDataTypeStr=Inherit: Same as second input
  Sum : Sum  Inputs=|++
  Sum1 : Sum  Inputs=|+-
  Sum2 : Sum  Inputs=+-|
  Sum3 : Sum  Inputs=|++
  Sum4 : Sum  Inputs=++-
  Sum5 : Sum  Inputs=+++
  Transfer Fcn2 : TransferFcn  Denominator=[0.005 1]
  Transfer Fcn3 : TransferFcn  Denominator=[0.005 1]
  d-axis-control : Scope  NumInputPorts=3
  q-axis control : Scope  NumInputPorts=3
  Out1 : Outport
  wires:
  Mux/1 -> Out1/1
  Gain/1 -> Sum/1
  Integrator1/1 -> Sum/2
  Gain1/1 -> Integrator1/1
  Sum1/1 -> d-axis-control/1, PID Controller1/1, Gain/1, Gain1/1
  ref/1 -> Demux/1
  meas/1 -> Demux1/1
  Demux1/2 -> Sum2/2, Gain5/1
  Demux1/1 -> Gain4/1, Sum1/2
  Demux/2 -> Sum2/1
  Demux/1 -> Sum1/1
  PID Controller/1 -> Mux2/2, Sum5/2
  Gain3/1 -> Integrator2/1
  Integrator2/1 -> Sum3/2
  Gain2/1 -> Sum3/1
  Sum2/1 -> PID Controller/1, q-axis control/1, Gain3/1, Gain2/1
  Sum4/1 -> d-axis-control/3, Mux/1
  Gain5/1 -> Mux1/3, Sum4/3
  Gain4/1 -> Mux2/3, Sum5/1
  Demux2/2 -> Transfer Fcn3/1
  Sum5/1 -> q-axis control/3, Mux/2
  V grid meas/1 -> Demux2/1
  Demux2/1 -> Transfer Fcn2/1
  Transfer Fcn2/1 -> Mux1/1, Sum4/1
  Mux1/1 -> d-axis-control/2
  Mux2/1 -> q-axis control/2
  Transfer Fcn3/1 -> Mux2/1, Sum5/3
  PID Controller1/1 -> Mux1/2, Sum4/2

== system IdealGen_load_CtrlGen_wWT_abc_detailed/DC Link ==
  Current Measurement1 : spsCurrentMeasurementLib/Current Measurement  PhasorSimulation=off  OutputType=Complex  PSBequivalent=0
  DC-Link : Scope  NumInputPorts=2
  Series RLC Branch : spsSeriesRLCBranchLib/Series RLC Branch  LConnTagsString=__new0  RConnTagsString=__new0  BranchType=C  Resistance=1  Inductance=1e-3  SetiL0=off  InitialCurrent=0  Capacitance=C_dc/2  Setx0=on  InitialVoltage=V_dc/2  Measurements=None
  Series RLC Branch1 : spsSeriesRLCBranchLib/Series RLC Branch  LConnTagsString=__new0  RConnTagsString=__new0  BranchType=C  Resistance=1  Inductance=1e-3  SetiL0=off  InitialCurrent=0  Capacitance=C_dc/2  Setx0=on  InitialVoltage=V_dc/2  Measurements=None
  Voltage Measurement1 : spsVoltageMeasurementLib/Voltage Measurement  PhasorSimulation=off  OutputType=Complex  PSBequivalent=0
  + : PMIOPort  Side=Left
  - : PMIOPort  Port=2  Side=Left
  pos : PMIOPort  Port=3  Side=Right
  neg : PMIOPort  Port=4  Side=Right
  wires:
  Voltage Measurement1/1 -> DC-Link/1
  Current Measurement1/1 -> DC-Link/2
  connections:
  -/RConn1 -- Series RLC Branch1/RConn1 -- neg/RConn1 -- Voltage Measurement1/LConn2
  Series RLC Branch1/LConn1 -- Series RLC Branch/RConn1
  pos/RConn1 -- Current Measurement1/LConn1 -- +/RConn1 -- Voltage Measurement1/LConn1
  Series RLC Branch/LConn1 -- Current Measurement1/RConn1

== system IdealGen_load_CtrlGen_wWT_abc_detailed/DC init ==
  init : Inport
  second : Inport  Port=2
  Clock : Clock
  Switch : Switch  Criteria=u2 > Threshold  Threshold=1  SaturateOnIntegerOverflow=off  InputSameDT=off
  "   " : Outport
  wires:
  second/1 -> Switch/1
  init/1 -> Switch/3
  Clock/1 -> Switch/2
  Switch/1 -> "   "/1

== system IdealGen_load_CtrlGen_wWT_abc_detailed/DC init2 ==
  second : Inport
  init : Inport  Port=2
  Clock : Clock
  Switch : Switch  Criteria=u2 > Threshold  Threshold=2  SaturateOnIntegerOverflow=off  InputSameDT=off
  "   " : Outport
  wires:
  Switch/1 -> "   "/1
  Clock/1 -> Switch/2
  init/1 -> Switch/3
  second/1 -> Switch/1

== system IdealGen_load_CtrlGen_wWT_abc_detailed/DC init3 ==
  init : Inport
  second : Inport  Port=2
  Clock : Clock
  Switch : Switch  Criteria=u2 > Threshold  Threshold=1  SaturateOnIntegerOverflow=off  InputSameDT=off
  "   " : Outport
  wires:
  second/1 -> Switch/1
  init/1 -> Switch/3
  Clock/1 -> Switch/2
  Switch/1 -> "   "/1

== system IdealGen_load_CtrlGen_wWT_abc_detailed/DC init4 ==
  init : Inport
  second : Inport  Port=2
  Clock : Clock
  Switch : Switch  Criteria=u2 > Threshold  Threshold=1  SaturateOnIntegerOverflow=off  InputSameDT=off
  "   " : Outport
  wires:
  Switch/1 -> "   "/1
  Clock/1 -> Switch/2
  init/1 -> Switch/3
  second/1 -> Switch/1

== system IdealGen_load_CtrlGen_wWT_abc_detailed/DC init5 ==
  init : Inport
  second : Inport  Port=2
  Clock : Clock
  Switch : Switch  Criteria=u2 > Threshold  Threshold=1  SaturateOnIntegerOverflow=off  InputSameDT=off
  "   " : Outport
  wires:
  Switch/1 -> "   "/1
  Clock/1 -> Switch/2
  init/1 -> Switch/3
  second/1 -> Switch/1

== system IdealGen_load_CtrlGen_wWT_abc_detailed/DC-link voltage controller ==
  ref : Inport
  meas : Inport  Port=2
  Gain : Gain  Commented=through  Gain=-1
  Gain1 : Gain
  Mux : Mux  Inputs=2
  PID Controller : slpidlib/PID Controller  Controller=PI  Form=Parallel  TimeDomain=Continuous-time  UseExternalTs=off  SampleTime=-1  IntegratorMethod=Forward Euler  FilterMethod=Forward Euler  ControllerParametersSource=internal  P=5  I=0.05  UseKiTs=off  D=0  N=100  UseFilter=on  TunerSelectOption=Transfer Function Based (PID Tuner App)  InitialConditionSource=internal  InitialConditionForIntegrator=0  InitialConditionForFilter=0  DifferentiatorICPrevScaledInput=0  ExternalReset=none  TrackingMode=off  Kt=1  LimitOutput=off  SatLimitsSource=internal  UpperSaturationLimit=0.5  LowerSaturationLimit=-0.5  LinearizeAsGain=on  AntiWindupMode=clamping  Kb=1  LimitIntegrator=off  UpperIntegratorSaturationLimit=0.5  LowerIntegratorSaturationLimit=-0.5  POutMin=[]  POutMax=[]  IOutMin=[]  IOutMax=[]  DOutMin=[]  DOutMax=[]  NOutMin=[]  NOutMax=[]  SumOutMin=[]  SumOutMax=[]  SaturationOutMin=[]  SaturationOutMax=[]  PParamMin=[]  PParamMax=[]  IParamMin=[]  IParamMax=[]  DParamMin=[]  DParamMax=[]  NParamMin=[]  NParamMax=[]  KbParamMin=[]  KbParamMax=[]  KtParamMin=[]  KtParamMax=[]  KbOutMin=[]  KbOutMax=[]  KtOutMin=[]  KtOutMax=[]  IntegratorOutMin=[]  IntegratorOutMax=[]  FilterOutMin=[]  FilterOutMax=[]  SumI1OutMin=[]  SumI1OutMax=[]  SumI2OutMin=[]  SumI2OutMax=[]  SumI3OutMin=[]  SumI3OutMax=[]  SumI4OutMin=[]  SumI4OutMax=[]  SumDOutMin=[]  SumDOutMax=[]  DifferentiatorOutMin=[]  DifferentiatorOutMax=[]  FilterDiffOutCoefMin=[]  FilterDiffOutCoefMax=[]  ReciprocalOutMin=[]  ReciprocalOutMax=[]  SumDenOutMin=[]  SumDenOutMax=[]  SumNumOutMin=[]  SumNumOutMax=[]  DivideOutMin=[]  DivideOutMax=[]  UdiffTsProdOutMin=[]  UdiffTsProdOutMax=[]  NTsProdOutMin=[]  NTsProdOutMax=[]  UintegralTsProdOutMin=[]  UintegralTsProdOutMax=[]  UngainTsProdOutMin=[]  UngainTsProdOutMax=[]  ClampingZeroOutDataTypeStr=Inherit: Inherit via back propagation  ClampingZeroOutMin=[]  ClampingZeroOutMax=[]  FilterDenConstantOutDataTypeStr=Inherit: Inherit via back propagation  FilterDenConstantOutMin=[]  FilterDenConstantOutMax=[]  PCopyOutDataTypeStr=Inherit: Inherit via back propagation  PCopyOutMin=[]  PCopyOutMax=[]  NCopyOutDataTypeStr=Inherit: Inherit via back propagation  NCopyOutMin=[]  NCopyOutMax=[]  IntegratorContinuousStateAttributes=''  IntegratorStateMustResolveToSignalObject=off  IntegratorRTWStateStorageClass=Auto  FilterContinuousStateAttributes=''  FilterStateMustResolveToSignalObject=off  FilterRTWStateStorageClass=Auto  ParallelPVariant=InternalParameters  IdealPVariant=Disabled  IVariant=InternalParameters  DVariant=Disabled  IntegratorVariant=Continuous  SatVariant=Disabled  AWVariant=Passthrough  PCopyVariant=Disabled  TRVariant=Disabled  FdbkBlocksVariant=Forward  IdealPFdbkVariant=Disabled  SatFdbkVariant=Disabled  DerivativeFilterVariant=Disabled  NVariant=Disabled  NCopyVariant=Disabled_SignalSpec  FilterICVariant=Disabled  IntegratorICVariant=InternalICs  ExternalResetVariant=Disabled  TRSumVariant=Passthrough  SumFdbkVariant=Disabled  SumVariant=Sum_PI  TsampFilterVariant=InternalTs  TsampNgainVariant=Passthrough  TsampIntegralVariant=Disabled_SignalSpec  ExternalSaturationOutDataTypeStr=Inherit: Same as second input
  Sum : Sum  Inputs=+-|
  Transfer Fcn : TransferFcn  Numerator=[8]  Denominator=[1 4*0.707 8]
  input : Outport
  error : Outport  Port=2
  out : Outport  Port=3
  Out4 : Outport  Port=4
  wires:
  Mux/1 -> input/1
  PID Controller/1 -> out/1, Gain/1
  Gain/1 -> Out4/1
  Sum/1 -> error/1, PID Controller/1, Gain1/1
  Gain1/1 -> Transfer Fcn/1
  ref/1 -> Mux/1, Sum/1
  meas/1 -> Mux/2, Sum/2

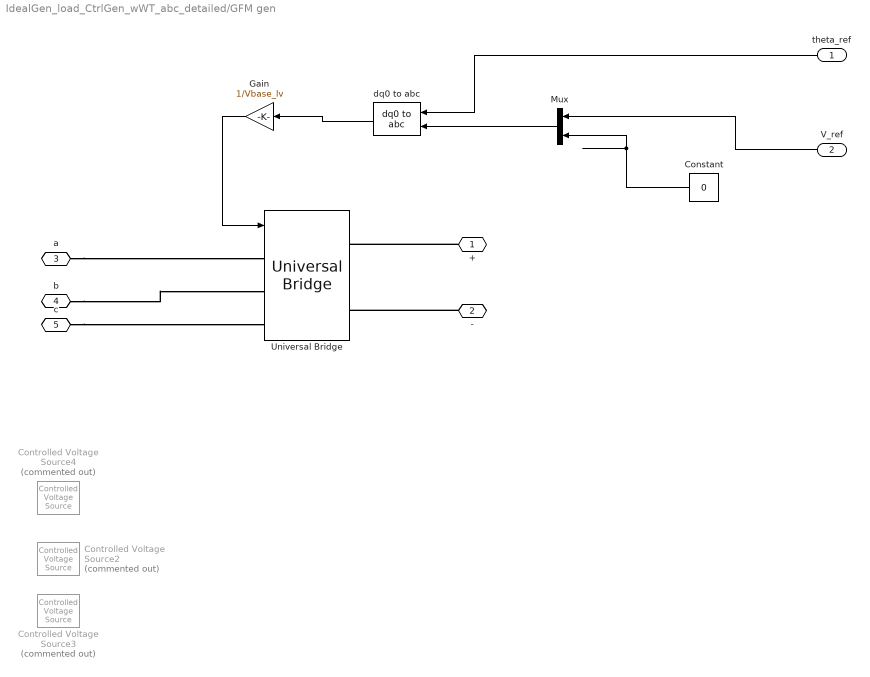
== system IdealGen_load_CtrlGen_wWT_abc_detailed/GFM gen ==
  theta_ref : Inport
  V_ref : Inport  Port=2
  Constant : Constant  Value=0
  Controlled Voltage Source2 : spsControlledVoltageSourceLib/Controlled Voltage Source  Commented=on  Initialize=on  Source_Type=AC  Amplitude=Vbase_lv  Phase=-120  Frequency=50  Measurements=None
  Controlled Voltage Source3 : spsControlledVoltageSourceLib/Controlled Voltage Source  Commented=on  Initialize=on  Source_Type=AC  Amplitude=Vbase_lv  Phase=120  Frequency=50  Measurements=None
  Controlled Voltage Source4 : spsControlledVoltageSourceLib/Controlled Voltage Source  Commented=on  Initialize=on  Source_Type=AC  Amplitude=Vbase_lv  Phase=0  Frequency=50  Measurements=None
  Gain : Gain  Gain=1/Vbase_lv
  Mux : Mux  Inputs=2
  Universal Bridge : spsUniversalBridgeLib/Universal Bridge  Arms=3  SnubberResistance=1e5  SnubberCapacitance=inf  Device=Average-model based VSC  Ron=1e-3  Lon=0  ForwardVoltages="[  0  0  ]"  ForwardVoltage=0  GTOparameters=[ 10e-6 , 20e-6 ]  IGBTparameters=[ 1e-6 , 2e-6 ]  Measurements=None  Measurements_2=None  converterType=Rectifier
  dq0 to abc : spsdq0toabcLib/dq0 to abc  Alignment=90 degrees behind phase A axis
  + : PMIOPort  Side=Left
  - : PMIOPort  Port=2  Side=Left
  a : PMIOPort  Port=3  Side=Right
  b : PMIOPort  Port=4  Side=Right
  c : PMIOPort  Port=5  Side=Right
  wires:
  Mux/1 -> dq0 to abc/1
  Constant/1 -> Mux/2
  dq0 to abc/1 -> Gain/1
  V_ref/1 -> Mux/1
  theta_ref/1 -> dq0 to abc/2
  Gain/1 -> Universal Bridge/1
  connections:
  c/RConn1 -- Universal Bridge/LConn3
  a/RConn1 -- Universal Bridge/LConn1
  b/RConn1 -- Universal Bridge/LConn2
  -/RConn1 -- Universal Bridge/RConn2
  +/RConn1 -- Universal Bridge/RConn1

== system IdealGen_load_CtrlGen_wWT_abc_detailed/Phase shifts ==
  From Workspace : FromWorkspace  Commented=on  VariableName=phase_shifts  OutputAfterFinalValue=Setting to zero
  Step : Step  Time=phase_shifts(1,1)  After=phase_shifts(1,2)  SampleTime=0
  Step1 : Step  Time=phase_shifts(2,1)  After=phase_shifts(2,2)  SampleTime=0
  Step2 : Step  Time=phase_shifts(3,1)  After=phase_shifts(3,2)  SampleTime=0
  Sum1 : Sum  Inputs=+++
  Out2 : Outport
  wires:
  Sum1/1 -> Out2/1
  Step/1 -> Sum1/1
  Step2/1 -> Sum1/3
  From Workspace/1 -> ?
  Step1/1 -> Sum1/2

== system IdealGen_load_CtrlGen_wWT_abc_detailed/ROCOF test ==
  Clock : Clock
  Constant4 : Constant  Value=0
  Constant5 : Constant
  Ramp : simulink/Sources/Ramp  slope=rocof_slope  start=Trocof_start  InitialOutput=0
  Sample and Hold : spsSampleandHoldLib/Sample and Hold  ic=0  Ts=0
      settings: LibrarySourceBlock=|
      | sps_lib/Control/Sample and
      | Hold
  Switch : Switch  Criteria=u2 > Threshold  Threshold=Trocof_start  SaturateOnIntegerOverflow=off  InputSameDT=off
  Switch1 : Switch  Threshold=Trocof_end  SaturateOnIntegerOverflow=off  InputSameDT=off
  Outport : Outport
  wires:
  Clock/1 -> Switch/2, Switch1/2
  Constant4/1 -> Switch/3, Switch1/1
  Sample and Hold/1 -> Outport/1
  Ramp/1 -> Switch/1
  Constant5/1 -> Switch1/3
  Switch/1 -> Sample and Hold/1
  Switch1/1 -> Sample and Hold/2

== system IdealGen_load_CtrlGen_wWT_abc_detailed/Subsystem ==
  note: Circular Current limiter
  In1 : Inport
  Abs : Abs
  Constant10 : Constant
  Constant9 : Constant  Value=1.2
  Demux4 : Demux  Outputs=2
  First-Order Filter1 : spsFirstOrderFilterLib/First-Order Filter  FilterType=Lowpass  Tc=0.002  Ts=0  Initialize=on  Vac_Init=[0, 0, 60]  Vdc_Init=0  PlotResponse=off  FreqRange="[0,  200,  1]"
  GreaterThan : RelationalOperator  Operator=>  OutDataTypeStr=boolean  RndMeth=Simplest  InputSameDT=off
  I_d_error5 : Scope
  I_d_error7 : Scope
  Kip6 : Gain
  Kip9 : Gain  Gain=1/1.2
  Real-Imag to Complex : RealImagToComplex
  Switch2 : Switch  Threshold=1  SaturateOnIntegerOverflow=off  InputSameDT=off
  Unit Delay6 : UnitDelay  InitialCondition=30e3  SampleTime=-1  HasFrameUpgradeWarning=on
  Out1 : Outport
  wires:
  Constant9/1 -> GreaterThan/2
  Demux4/2 -> Real-Imag to Complex/2
  Kip9/1 -> Switch2/1
  In1/1 -> First-Order Filter1/1
  Real-Imag to Complex/1 -> Abs/1
  Abs/1 -> GreaterThan/1, I_d_error5/1, Kip9/1
  GreaterThan/1 -> Switch2/2
  Constant10/1 -> Switch2/3
  First-Order Filter1/1 -> Demux4/1
  Switch2/1 -> I_d_error7/1, Kip6/1
  Demux4/1 -> Real-Imag to Complex/1
  Kip6/1 -> Unit Delay6/1
  Unit Delay6/1 -> Out1/1

== system IdealGen_load_CtrlGen_wWT_abc_detailed/Subsystem1 ==
  In2 : Inport
  In1 : Inport  Port=2
  Sqrt : Sqrt
  Square : Math  Operator=square
  Square1 : Math  Operator=square
  Sum2 : Sum  Inputs=|++
  Out1 : Outport
  wires:
  Sum2/1 -> Sqrt/1
  Sqrt/1 -> Out1/1
  Square/1 -> Sum2/1
  In2/1 -> Square1/1
  Square1/1 -> Sum2/2
  In1/1 -> Square/1

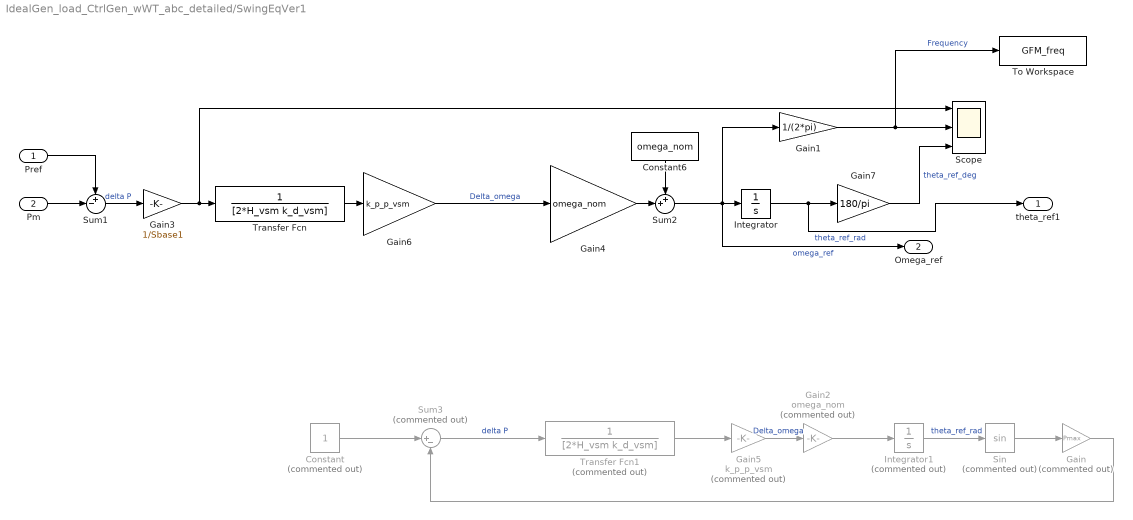
== system IdealGen_load_CtrlGen_wWT_abc_detailed/SwingEqVer1 ==
  Pref : Inport
  Pm : Inport  Port=2
  Constant : Constant  Commented=on
  Constant6 : Constant  Value=omega_nom
  Gain : Gain  Commented=on  Gain=Pmax
  Gain1 : Gain  Gain=1/(2*pi)
  Gain2 : Gain  Commented=on  Gain=omega_nom
  Gain3 : Gain  Gain=1/Sbase1
  Gain4 : Gain  Gain=omega_nom
  Gain5 : Gain  Commented=on  Gain=k_p_p_vsm
  Gain6 : Gain  Gain=k_p_p_vsm
  Gain7 : Gain  Gain=180/pi
  Integrator : Integrator  WrappedStateUpperValue=2*pi  WrappedStateLowerValue=0
  Integrator1 : Integrator  Commented=on  WrappedStateUpperValue=2*pi  WrappedStateLowerValue=0
  Scope : Scope  NumInputPorts=3
  Sin : Trigonometry  Commented=on
  Sum1 : Sum  Inputs=+-|
  Sum2 : Sum  Inputs=++|
  Sum3 : Sum  Commented=on  Inputs=|+-
  To Workspace : ToWorkspace  VariableName=GFM_freq  SaveFormat=Structure With Time  SampleTime=-1
  Transfer Fcn : TransferFcn  Denominator=[2*H_vsm k_d_vsm]
  Transfer Fcn1 : TransferFcn  Commented=on  Denominator=[2*H_vsm k_d_vsm]
  theta_ref1 : Outport
  Omega_ref : Outport  Port=2
  wires:
  Sum1/1 -> Gain3/1  "delta P"
  Integrator/1 -> theta_ref1/1, Gain7/1  "theta_ref_rad"
  Sum2/1 -> Gain1/1, Omega_ref/1, Integrator/1  "omega_ref"
  Transfer Fcn/1 -> Gain6/1
  Gain6/1 -> Gain4/1  "Delta_omega"
  Pm/1 -> Sum1/2
  Gain3/1 -> Scope/1, Transfer Fcn/1
  Gain7/1 -> Scope/3  "theta_ref_deg"
  Pref/1 -> Sum1/1
  Constant6/1 -> Sum2/1
  Gain4/1 -> Sum2/2
  Gain1/1 -> To Workspace/1, Scope/2  "Frequency"
  Gain5/1 -> Gain2/1  "Delta_omega"
  Transfer Fcn1/1 -> Gain5/1
  Sum3/1 -> Transfer Fcn1/1  "delta P"
  Gain2/1 -> Integrator1/1
  Sin/1 -> Gain/1
  Gain/1 -> Sum3/2
  Constant/1 -> Sum3/1
  Integrator1/1 -> Sin/1  "theta_ref_rad"

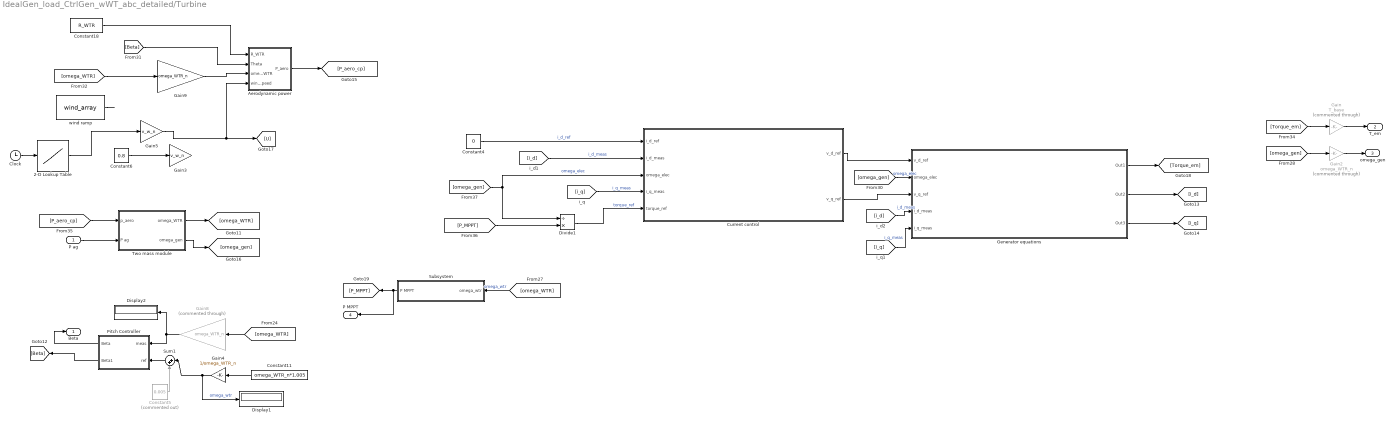
== system IdealGen_load_CtrlGen_wWT_abc_detailed/Turbine ==
  P ag : Inport
  2-D Lookup Table : Lookup_n-D  NumberOfTableDimensions=1  BreakpointsForDimension1=wind_array_step(1,:)  BreakpointsForDimension2=[1:3]  IndexSearchMethod=Linear search  Table=wind_array_step(2,:)  InterpMethod=Nearest  InternalRulePriority=Speed  RndMeth=Simplest
  Aerodynamic power : Subsystem
  Clock : Clock
  Constant11 : Constant  Value=omega_WTR_n*1.005
  Constant18 : Constant  Value=R_WTR
  Constant4 : Constant  Value=0
  Constant5 : Constant  Commented=on  Value=0.005
  Constant6 : Constant  Value=0.8
  Current control : Subsystem
  Display1 : Display
  Display2 : Display
  Divide1 : Product  Inputs=/*
  Gain : Gain  Commented=through  Gain=T_base
  Gain2 : Gain  Commented=through  Gain=omega_WTR_n
  Gain3 : Gain  Gain=v_w_n
  Gain4 : Gain  Gain=1/omega_WTR_n
  Gain5 : Gain  Gain=v_w_n
  Gain8 : Gain  Commented=through  Gain=omega_WTR_n
  Gain9 : Gain  Gain=omega_WTR_n
  Generator equations : Subsystem
  Pitch Controller : Subsystem
  Subsystem : Subsystem
  Sum1 : Sum  Inputs=|++
  Two mass module : Subsystem
  wind ramp : FromWorkspace  VariableName=wind_array
  Beta : Outport
  T_em : Outport  Port=2
  omega_gen : Outport  Port=3
  P MPPT : Outport  Port=4
  wires:
  [omega_gen] -> Gain2/1
  [omega_WTR] -> Subsystem/1(omega_wtr)  "omega_wtr"
  [i_d] -> Current control/2(i_d_meas)  "i_d_meas"
  Generator equations/3(Out3) -> [i_q]
  [i_q] -> Generator equations/5(i_q_meas)  "i_q_meas"
  Pitch Controller/1(Beta) -> Beta/1
  [i_d] -> Generator equations/4(i_d_meas)  "i_d_meas"
  Constant18/1 -> Aerodynamic power/1(R_WTR)
  [omega_gen] -> Generator equations/2(omega_elec)  "omega_elec"
  Gain5/1 -> Aerodynamic power/4(wind speed), [U]
  P ag/1 -> Two mass module/2(P ag)
  Constant11/1 -> Gain4/1
  wind ramp/1 -> ?
  [P_aero_cp] -> Two mass module/1(p_aero)
  Constant4/1 -> Current control/1(i_d_ref)  "i_d_ref"
  Generator equations/1(Out1) -> [Torque_em]
  Constant5/1 -> Sum1/2
  Two mass module/1(omega_WTR) -> [omega_WTR]
  [P_MPPT] -> Divide1/2
  Two mass module/2(omega_gen) -> [omega_gen]
  [omega_gen] -> Divide1/1, Current control/3(omega_elec)  "omega_elec"
  Sum1/1 -> Pitch Controller/2(ref)
  Gain4/1 -> Sum1/1, Display1/1  "omega_wtr"
  Constant6/1 -> Gain3/1
  [omega_WTR] -> Gain8/1
  Clock/1 -> 2-D Lookup Table/1
  Pitch Controller/2(Beta1) -> [Beta]
  [i_q] -> Current control/4(i_q_meas)  "i_q_meas"
  Aerodynamic power/1(P_aero) -> [P_aero_cp]
  Gain9/1 -> Aerodynamic power/3(omega_WTR)
  Gain8/1 -> Display2/1, Pitch Controller/1(meas)
  [Beta] -> Aerodynamic power/2(Theta)
  2-D Lookup Table/1 -> Gain5/1
  [Torque_em] -> Gain/1
  Subsystem/1(P MPPT) -> P MPPT/1, [P_MPPT]
  Divide1/1 -> Current control/5(torque_ref)  "torque_ref"
  Current control/1(v_d_ref) -> Generator equations/1(v_d_ref)
  Generator equations/2(Out2) -> [i_d]
  [omega_WTR] -> Gain9/1
  Current control/2(v_q_ref) -> Generator equations/3(v_q_ref)
  Gain/1 -> T_em/1
  Gain2/1 -> omega_gen/1
